simulink model "Simulink_speed_control_by_field_weakening_oldver"  (R2023b)
settings: Solver=VariableStepAuto  StartTime=0.0  StopTime=50  RelTol=1e-3
values from neighbouring files (symbols this model uses):
  J = 0.068    [DCmotor_speed_control_parameter.m]
  Ka = 1    [DCmotor_speed_control_parameter.m]
  La = 2.3e-3    (= 0.0023)    [DCmotor_speed_control_parameter.m]
  M = 1.304    [DCmotor_speed_control_parameter.m]
  R_f = 356.7    [DCmotor_speed_control_parameter.m]
  Ra = 0.3    [DCmotor_speed_control_parameter.m]
  speed_ref = 20    [DCmotor_speed_control_parameter.m]
  Tload = 0    [DCmotor_speed_control_parameter.m]
undefined symbols (not defined in the file or in its folder): i_a_rated, Pmax, v_f_rated, v_t_rated
libraries: slpidlib x2
settings Model: Creator=chayutht  LastModifiedBy=chayutht

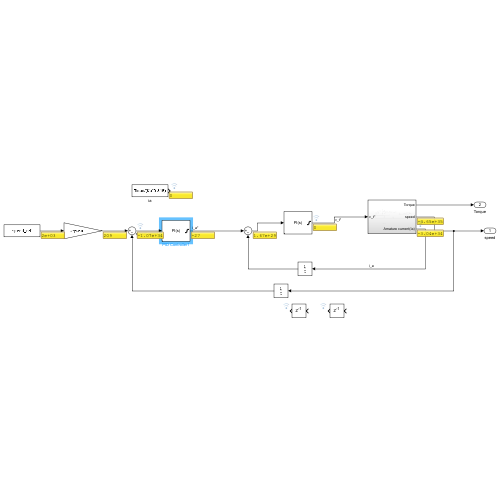
[thumbnail: Simulink's stored preview of the top-level diagram]
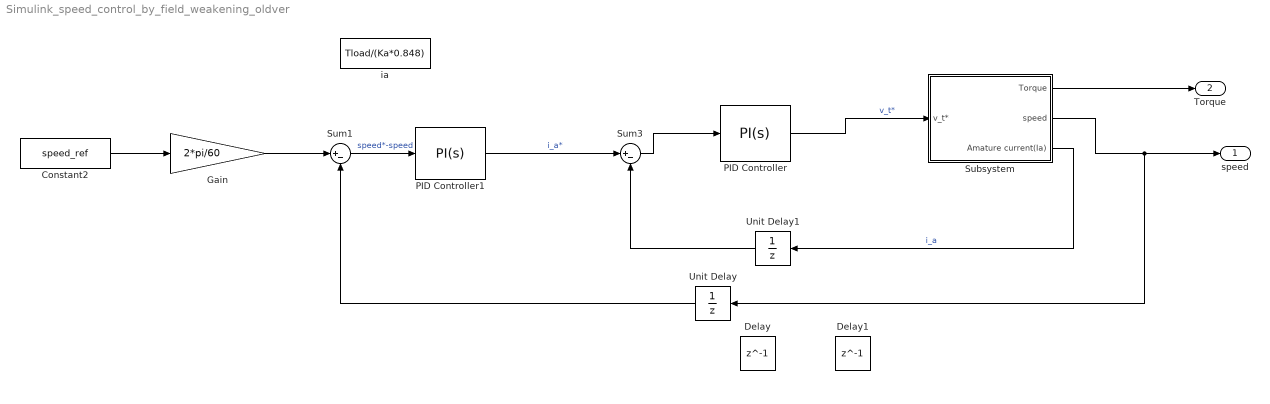
== system Simulink_speed_control_by_field_weakening_oldver ==
  Constant2 : Constant  Value=speed_ref
  Delay : Delay  DelayLength=1  InitialCondition=0
  Delay1 : Delay  DelayLength=1  InitialCondition=0
  Gain : Gain  Gain=2*pi/60
  PID Controller : slpidlib/PID Controller  Controller=PI  Form=Parallel  TimeDomain=Continuous-time  UseExternalTs=off  SampleTime=-1  IntegratorMethod=Forward Euler  FilterMethod=Forward Euler  ControllerParametersSource=internal  P=0.1  I=5  UseKiTs=off  D=0  N=100  UseFilter=on  TunerSelectOption=Frequency Response Based  InitialConditionSource=internal  InitialConditionForIntegrator=0  InitialConditionForFilter=0  DifferentiatorICPrevScaledInput=0  ExternalReset=none  TrackingMode=off  Kt=1  LimitOutput=on  SatLimitsSource=internal  UpperSaturationLimit=v_t_rated  LowerSaturationLimit=0  LinearizeAsGain=on  AntiWindupMode=none  Kb=1  LimitIntegrator=off  UpperIntegratorSaturationLimit=inf  LowerIntegratorSaturationLimit=-inf  POutMin=[]  POutMax=[]  IOutMin=[]  IOutMax=[]  DOutMin=[]  DOutMax=[]  NOutMin=[]  NOutMax=[]  SumOutMin=[]  SumOutMax=[]  SaturationOutMin=[]  SaturationOutMax=[]  PParamMin=[]  PParamMax=[]  IParamMin=[]  IParamMax=[]  DParamMin=[]  DParamMax=[]  NParamMin=[]  NParamMax=[]  KbParamMin=[]  KbParamMax=[]  KtParamMin=[]  KtParamMax=[]  KbOutMin=[]  KbOutMax=[]  KtOutMin=[]  KtOutMax=[]  IntegratorOutMin=[]  IntegratorOutMax=[]  FilterOutMin=[]  FilterOutMax=[]  SumI1OutMin=[]  SumI1OutMax=[]  SumI2OutMin=[]  SumI2OutMax=[]  SumI3OutMin=[]  SumI3OutMax=[]  SumI4OutMin=[]  SumI4OutMax=[]  SumDOutMin=[]  SumDOutMax=[]  DifferentiatorOutMin=[]  DifferentiatorOutMax=[]  FilterDiffOutCoefMin=[]  FilterDiffOutCoefMax=[]  ReciprocalOutMin=[]  ReciprocalOutMax=[]  SumDenOutMin=[]  SumDenOutMax=[]  SumNumOutMin=[]  SumNumOutMax=[]  DivideOutMin=[]  DivideOutMax=[]  UdiffTsProdOutMin=[]  UdiffTsProdOutMax=[]  NTsProdOutMin=[]  NTsProdOutMax=[]  UintegralTsProdOutMin=[]  UintegralTsProdOutMax=[]  UngainTsProdOutMin=[]  UngainTsProdOutMax=[]  ClampingZeroOutDataTypeStr=Inherit: Inherit via back propagation  ClampingZeroOutMin=[]  ClampingZeroOutMax=[]  FilterDenConstantOutDataTypeStr=Inherit: Inherit via back propagation  FilterDenConstantOutMin=[]  FilterDenConstantOutMax=[]  PCopyOutDataTypeStr=Inherit: Inherit via back propagation  PCopyOutMin=[]  PCopyOutMax=[]  NCopyOutDataTypeStr=Inherit: Inherit via back propagation  NCopyOutMin=[]  NCopyOutMax=[]  IntegratorContinuousStateAttributes=''  IntegratorStateMustResolveToSignalObject=off  IntegratorRTWStateStorageClass=Auto  FilterContinuousStateAttributes=''  FilterStateMustResolveToSignalObject=off  FilterRTWStateStorageClass=Auto  ParallelPVariant=InternalParameters  IdealPVariant=Disabled  IVariant=InternalParameters  DVariant=Disabled  IntegratorVariant=Continuous  SatVariant=Enabled  AWVariant=Passthrough  PCopyVariant=Disabled  TRVariant=Disabled  FdbkBlocksVariant=Forward  IdealPFdbkVariant=Disabled  SatFdbkVariant=Disabled  DerivativeFilterVariant=Disabled  NVariant=Disabled  NCopyVariant=Disabled_SignalSpec  FilterICVariant=Disabled  IntegratorICVariant=InternalICs  ExternalResetVariant=Disabled  TRSumVariant=Passthrough  SumFdbkVariant=Disabled  SumVariant=Sum_PI  TsampFilterVariant=InternalTs  TsampNgainVariant=Passthrough  TsampIntegralVariant=Disabled_SignalSpec  ExternalSaturationOutDataTypeStr=Inherit: Same as second input
  PID Controller1 : slpidlib/PID Controller  Controller=PI  Form=Parallel  TimeDomain=Continuous-time  UseExternalTs=off  SampleTime=-1  IntegratorMethod=Forward Euler  FilterMethod=Forward Euler  ControllerParametersSource=internal  P=0.1  I=1  UseKiTs=off  D=0.1  N=100  UseFilter=on  TunerSelectOption=Transfer Function Based (PID Tuner App)  InitialConditionSource=internal  InitialConditionForIntegrator=0  InitialConditionForFilter=0  DifferentiatorICPrevScaledInput=0  ExternalReset=none  TrackingMode=off  Kt=1  LimitOutput=on  SatLimitsSource=internal  UpperSaturationLimit=i_a_rated  LowerSaturationLimit=-i_a_rated  LinearizeAsGain=on  AntiWindupMode=none  Kb=1  LimitIntegrator=off  UpperIntegratorSaturationLimit=inf  LowerIntegratorSaturationLimit=-inf  POutMin=[]  POutMax=[]  IOutMin=[]  IOutMax=[]  DOutMin=[]  DOutMax=[]  NOutMin=[]  NOutMax=[]  SumOutMin=[]  SumOutMax=[]  SaturationOutMin=[]  SaturationOutMax=[]  PParamMin=[]  PParamMax=[]  IParamMin=[]  IParamMax=[]  DParamMin=[]  DParamMax=[]  NParamMin=[]  NParamMax=[]  KbParamMin=[]  KbParamMax=[]  KtParamMin=[]  KtParamMax=[]  KbOutMin=[]  KbOutMax=[]  KtOutMin=[]  KtOutMax=[]  IntegratorOutMin=[]  IntegratorOutMax=[]  FilterOutMin=[]  FilterOutMax=[]  SumI1OutMin=[]  SumI1OutMax=[]  SumI2OutMin=[]  SumI2OutMax=[]  SumI3OutMin=[]  SumI3OutMax=[]  SumI4OutMin=[]  SumI4OutMax=[]  SumDOutMin=[]  SumDOutMax=[]  DifferentiatorOutMin=[]  DifferentiatorOutMax=[]  FilterDiffOutCoefMin=[]  FilterDiffOutCoefMax=[]  ReciprocalOutMin=[]  ReciprocalOutMax=[]  SumDenOutMin=[]  SumDenOutMax=[]  SumNumOutMin=[]  SumNumOutMax=[]  DivideOutMin=[]  DivideOutMax=[]  UdiffTsProdOutMin=[]  UdiffTsProdOutMax=[]  NTsProdOutMin=[]  NTsProdOutMax=[]  UintegralTsProdOutMin=[]  UintegralTsProdOutMax=[]  UngainTsProdOutMin=[]  UngainTsProdOutMax=[]  ClampingZeroOutDataTypeStr=Inherit: Inherit via back propagation  ClampingZeroOutMin=[]  ClampingZeroOutMax=[]  FilterDenConstantOutDataTypeStr=Inherit: Inherit via back propagation  FilterDenConstantOutMin=[]  FilterDenConstantOutMax=[]  PCopyOutDataTypeStr=Inherit: Inherit via back propagation  PCopyOutMin=[]  PCopyOutMax=[]  NCopyOutDataTypeStr=Inherit: Inherit via back propagation  NCopyOutMin=[]  NCopyOutMax=[]  IntegratorContinuousStateAttributes=''  IntegratorStateMustResolveToSignalObject=off  IntegratorRTWStateStorageClass=Auto  FilterContinuousStateAttributes=''  FilterStateMustResolveToSignalObject=off  FilterRTWStateStorageClass=Auto  ParallelPVariant=InternalParameters  IdealPVariant=Disabled  IVariant=InternalParameters  DVariant=Disabled  IntegratorVariant=Continuous  SatVariant=Enabled  AWVariant=Passthrough  PCopyVariant=Disabled  TRVariant=Disabled  FdbkBlocksVariant=Forward  IdealPFdbkVariant=Disabled  SatFdbkVariant=Disabled  DerivativeFilterVariant=Disabled  NVariant=Disabled  NCopyVariant=Disabled_SignalSpec  FilterICVariant=Disabled  IntegratorICVariant=InternalICs  ExternalResetVariant=Disabled  TRSumVariant=Passthrough  SumFdbkVariant=Disabled  SumVariant=Sum_PI  TsampFilterVariant=InternalTs  TsampNgainVariant=Passthrough  TsampIntegralVariant=Disabled_SignalSpec  ExternalSaturationOutDataTypeStr=Inherit: Same as second input
  Subsystem : Subsystem
  Sum1 : Sum  Inputs=|+-
  Sum3 : Sum  Inputs=|+-
  Unit Delay : UnitDelay  SampleTime=-1  HasFrameUpgradeWarning=on
  Unit Delay1 : UnitDelay  SampleTime=-1  HasFrameUpgradeWarning=on
  ia : Constant  Value=Tload/(Ka*0.848)
  speed : Outport
  Torque : Outport  Port=2
  wires:
  Sum3/1 -> PID Controller/1
  PID Controller/1 -> Subsystem/1(v_t*)  "v_t*"
  Subsystem/1(Torque) -> Torque/1
  Subsystem/2(speed) -> Unit Delay/1, speed/1
  Subsystem/3(Amature current(Ia)) -> Unit Delay1/1  "i_a"
  PID Controller1/1 -> Sum3/1  "i_a*"
  Sum1/1 -> PID Controller1/1  "speed*-speed"
  Constant2/1 -> Gain/1
  Gain/1 -> Sum1/1
  Unit Delay1/1 -> Sum3/2
  Unit Delay/1 -> Sum1/2

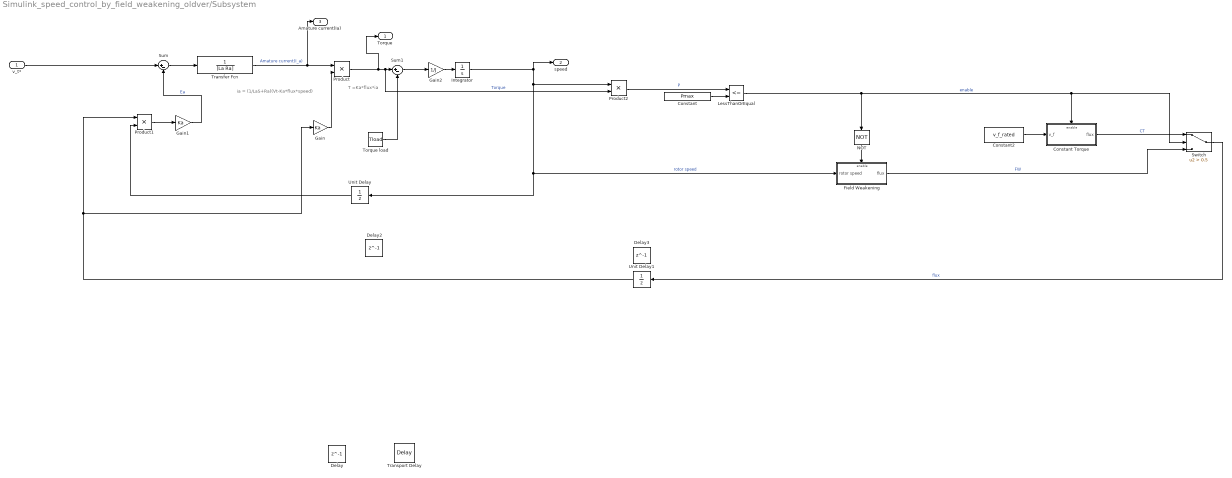
== system Simulink_speed_control_by_field_weakening_oldver/Subsystem ==
  note: T =Ka*flux*ia
  note: ia = (1/LaS+Ra)(Vt-Ka*flux*speed)
  v_t* : Inport
  Constant : Constant  Value=Pmax
  Constant Torque : Subsystem  TreatAsAtomicUnit=on
  Constant2 : Constant  Value=v_f_rated
  Delay : Delay  DelayLength=1  InitialCondition=0
  Delay2 : Delay  DelayLength=1  InitialCondition=0
  Delay3 : Delay  DelayLength=1  InitialCondition=0
  Field Weakening : Subsystem  TreatAsAtomicUnit=on
  Gain : Gain  Gain=Ka
  Gain1 : Gain  Gain=Ka
  Gain2 : Gain  Gain=1/J
  Integrator : Integrator  InitialCondition=500*2*pi/60
  LessThanOrEqual : RelationalOperator  Operator=<=  OutDataTypeStr=boolean  RndMeth=Simplest  InputSameDT=off
  NOT : Logic  Operator=NOT  IconShape=distinctive  AllPortsSameDT=off  OutDataTypeStr=boolean
  Product : Product
  Product1 : Product
  Product2 : Product
  Sum : Sum  Inputs=|+-
  Sum1 : Sum  Inputs=|+-
  Switch : Switch  Criteria=u2 > Threshold  Threshold=0.5  SaturateOnIntegerOverflow=off  InputSameDT=off
  Torque load : Constant  Value=Tload
  Transfer Fcn : TransferFcn  Denominator=[La Ra]
      settings: AttributesFormatString=%<Denominator>=(0.5 1)
  Transport Delay : TransportDelay  DelayTime=0.001
  Unit Delay : UnitDelay  SampleTime=-1  HasFrameUpgradeWarning=on
  Unit Delay1 : UnitDelay  SampleTime=-1  HasFrameUpgradeWarning=on
  Torque : Outport
  speed : Outport  Port=2
  Amature current(Ia) : Outport  Port=3
  wires:
  Gain/1 -> Product/2
  Integrator/1 -> speed/1, Unit Delay/1, Field Weakening/1(rotor speed), Product2/1  "rotor speed"
  Torque load/1 -> Sum1/2
  Sum1/1 -> Gain2/1
  v_t*/1 -> Sum/1
  Product/1 -> Product2/2, Sum1/1, Torque/1  "Torque"
  Gain2/1 -> Integrator/1
  Gain1/1 -> Sum/2  "Ea"
  Product1/1 -> Gain1/1
  Transfer Fcn/1 -> Amature current(Ia)/1, Product/1  "Amature current(I_a)"
  Sum/1 -> Transfer Fcn/1
  Switch/1 -> Unit Delay1/1  "flux"
  Constant/1 -> LessThanOrEqual/2
  Constant Torque/1(flux) -> Switch/1  "CT"
  Field Weakening/1(flux) -> Switch/3  "FW"
  Constant2/1 -> Constant Torque/1(v_f)
  Product2/1 -> LessThanOrEqual/1  "P"
  LessThanOrEqual/1 -> Switch/2, Constant Torque/Enable, NOT/1  "enable"
  NOT/1 -> Field Weakening/Enable
  Unit Delay/1 -> Product1/2
  Unit Delay1/1 -> Gain/1, Product1/1

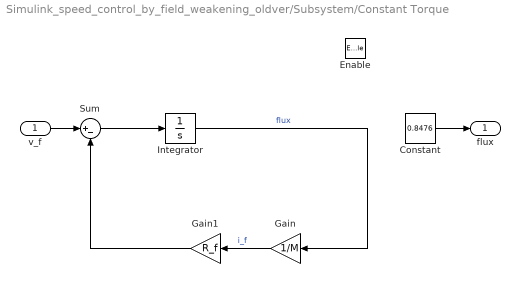
== system Simulink_speed_control_by_field_weakening_oldver/Subsystem/Constant Torque ==
  v_f : Inport
  Enable : EnablePort
  Constant : Constant  Value=0.8476
  Gain : Gain  Gain=1/M
  Gain1 : Gain  Gain=R_f
  Integrator : Integrator  InitialCondition=0.8476
  Sum : Sum  Inputs=|+-
  flux : Outport
  wires:
  v_f/1 -> Sum/1
  Sum/1 -> Integrator/1
  Integrator/1 -> Gain/1  "flux"
  Gain/1 -> Gain1/1  "i_f"
  Gain1/1 -> Sum/2
  Constant/1 -> flux/1

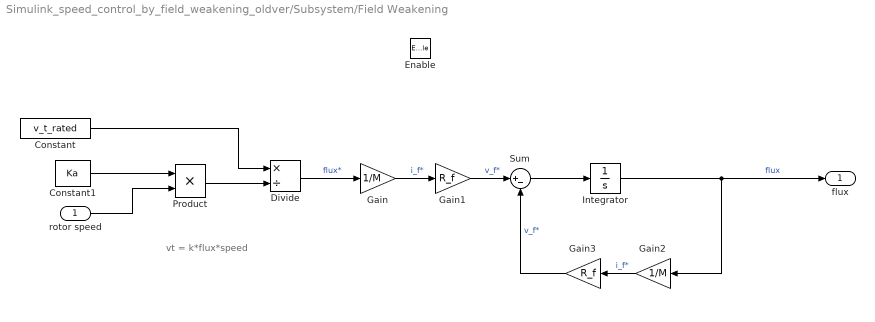
== system Simulink_speed_control_by_field_weakening_oldver/Subsystem/Field Weakening ==
  note: vt = k*flux*speed
  rotor speed : Inport
  Enable : EnablePort
  Constant : Constant  Value=v_t_rated
  Constant1 : Constant  Value=Ka
  Divide : Product  Inputs=*/
  Gain : Gain  Gain=1/M
  Gain1 : Gain  Gain=R_f
  Gain2 : Gain  Gain=1/M
  Gain3 : Gain  Gain=R_f
  Integrator : Integrator  InitialCondition=0.848
  Product : Product
  Sum : Sum  Inputs=|+-
  flux : Outport
  wires:
  Constant1/1 -> Product/1
  rotor speed/1 -> Product/2
  Product/1 -> Divide/2
  Constant/1 -> Divide/1
  Divide/1 -> Gain/1  "flux*"
  Gain/1 -> Gain1/1  "i_f*"
  Gain1/1 -> Sum/1  "v_f*"
  Sum/1 -> Integrator/1
  Integrator/1 -> Gain2/1, flux/1  "flux"
  Gain2/1 -> Gain3/1  "i_f*"
  Gain3/1 -> Sum/2  "v_f*"
